simulink model "mymodeltest"  (Simulink 8.3)
settings: Solver=ode45  StartTime=0.0  StopTime=5  RelTol=1e-3
settings Model: Creator=Ali  LastModifiedBy=Ali
settings DataIOCC: SignalLoggingSaveFormat=Dataset
settings DebuggingCC: UnderspecifiedInitializationDetection=Simplified  StateNameClashWarn=none
settings GRTTargetCC: CombineOutputUpdateFcns=on  GRTInterface=off

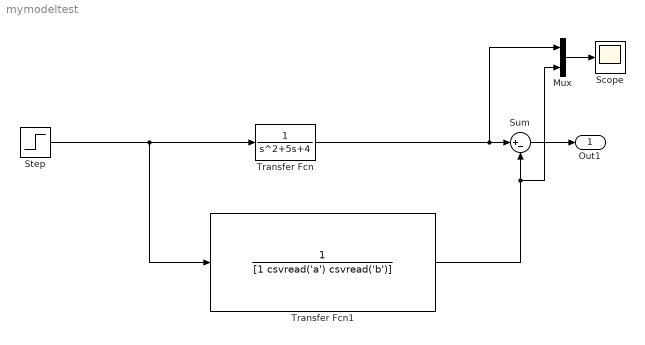
== system mymodeltest ==
  Mux : Mux  Inputs=2
  Scope : Scope
  Step : Step  SampleTime=0
  Sum : Sum  Inputs=|+-
  Transfer Fcn : TransferFcn  Denominator="[1  5  4]"
  Transfer Fcn1 : TransferFcn  Denominator=[1 csvread('a') csvread('b')]
  Out1 : Outport
  wires:
  Step/1 -> Transfer Fcn1/1, Transfer Fcn/1
  Transfer Fcn/1 -> Mux/1, Sum/1
  Transfer Fcn1/1 -> Mux/2, Sum/2
  Sum/1 -> Out1/1
  Mux/1 -> Scope/1
